simulink model "HEV_Simu_V1_1b"  (R2018a)
settings: Solver=ode23s  StartTime=0.0  StopTime=660  FixedStep=0.001  EnableMultiTasking=on
PreLoadFcn:
  | HevSimuVccWs_V1_PreLoad
  | %プラントモデルのコールバック・プリロード関数のバス定義
  | HEVPlant_Ptbs_V1_BusInfo
  | Engine_MapMdl_Ptbs_V1_BusInfo
  | Motor_MapMdl_Ptbs_V1_BusInfo
StartFcn:
  | tic
StopFcn:
  | toc
  | disp(['実時間の' num2str(max(tout)/toc) '倍速'])
model workspace (MAT data in the model file):
  Var = 0
undefined symbols (not defined in the file or in its folder): canChannel
libraries: canmsglib x108, canlib x35, simulink x2
(part 6 of 8)

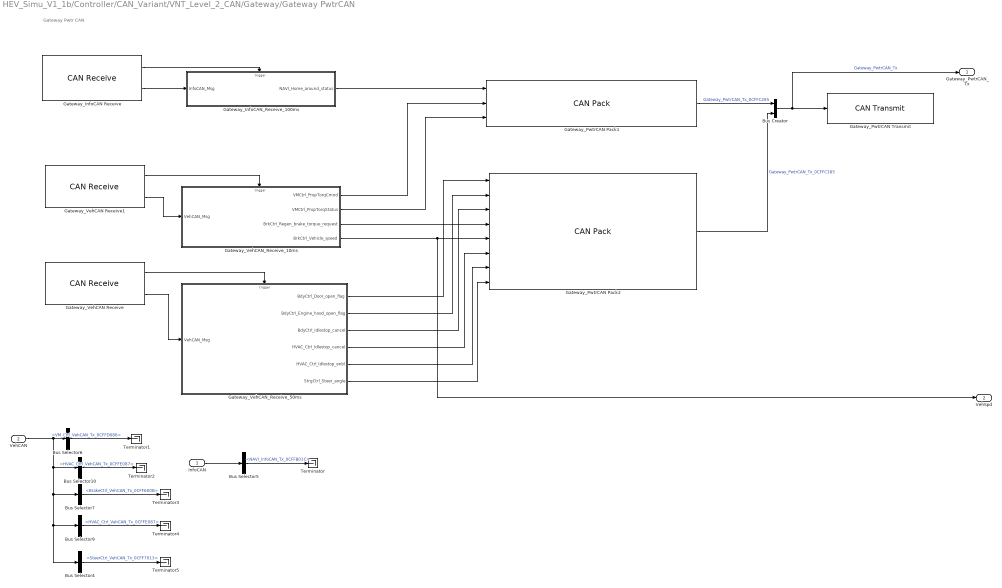
== system HEV_Simu_V1_1b/Controller/CAN_Variant/VNT_Level_2_CAN/Gateway/Gateway PwtrCAN ==
  note: Gateway Pwtr CAN
  InfoCAN : Inport
  VehCAN : Inport  Port=2
  Bus Creator : BusCreator  Inputs=2
  Bus Selector10 : BusSelector  OutputSignals=HVAC_Ctrl_VehCAN_Tx_0CFFE087
  Bus Selector4 : BusSelector  OutputSignals=SteerCtrl_VehCAN_Tx_0CFF7013
  Bus Selector5 : BusSelector  OutputSignals=NAVI_InfoCAN_Tx_0CFFB01C
  Bus Selector6 : BusSelector  OutputSignals=VM_Ctrl_VehCAN_Tx_0CFFD086
  Bus Selector7 : BusSelector  OutputSignals=BrakeCtrl_VehCAN_Tx_0CFF600B
  Bus Selector9 : BusSelector  OutputSignals=HVAC_Ctrl_VehCAN_Tx_0CFFE087
  Gateway_InfoCAN Receive : canlib/CAN Receive  BlockHandle=676.0001  DeviceMenu=MathWorks Virtual 1 (Channel 1)  Device=MathWorks Virtual 1 (Channel 1)  ObjConstructor=canChannel('MathWorks','Virtual 1',1)  EnableStandardIDsFilter=off  StandardIDs=0  EnableExtendedIDsFilter=off  ExtendedIDs=0  SampleTime=0.1  MsgsPerTimestep=all  StdIDsCombo=Allow all  ExtIDsCombo=Allow all  InternalFilterUpdateStatus=on  BusOutput=off
      settings: AttributesFormatString=<SampleTime = %<SampleTime>>  SourceProductName=Vehicle Network Toolbox  SourceProductBaseCode=VN
  Gateway_InfoCAN_Receive_100ms : Subsystem
  Gateway_PwtrCAN Pack1 : canmsglib/CAN Pack  CANdbFile=HEV_CANDB.dbc  MsgList=Gateway_PwtrCAN_Tx_1  MsgName=Gateway_PwtrCAN_Tx_1  MsgIDType=Extended (29-bit identifier)  MsgIdentifier=218088069  MsgLength=8  SignalInfo=NAVI_Home_around_status_G$0$16$1$2$1$0$1$0$0$65535$#VMCtrl_PropTorqCmnd_G$24$16$1$1$1$0$1.000000e-02$0$-300$300$#VMCtrl_PropTorqStatus_G$16$8$1$2$1$0$1$0$0$7$#  NSignals=3  StartBits=str2num('[int32(0);int32(24);int32(16)]')  SignalSizes=str2num('[int32(16);int32(16);int32(8)]')  ByteOrders=str2num('[int32(1);int32(1);int32(1)]')  DataTypes=str2num('[int32(2);int32(1);int32(2)]')  MultiplexTypes=str2num('[int32(1);int32(1);int32(1)]')  MultiplexValues=str2num('[double(0);double(0);double(0)]')  Factors=str2num('[double(1);double(1.000000e-02);double(1)]')  Offsets=str2num('[double(0);double(0);double(0)]')  Minimums=str2num('[double(0);double(-300);double(0)]')  Maximums=str2num('[double(65535);double(300);double(7)]')  Remote=off  ApplyMinMax=off  BusOutput=off
      settings: AttributesFormatString=<CANdbFile = %<CANdbFile>>  SourceProductName=Simulink Real-Time  SourceProductBaseCode=XP  DataFormat=CANdb specified signals
  Gateway_PwtrCAN Pack2 : canmsglib/CAN Pack  CANdbFile=HEV_CANDB.dbc  MsgList=Gateway_PwtrCAN_Tx_2  MsgName=Gateway_PwtrCAN_Tx_2  MsgIDType=Extended (29-bit identifier)  MsgIdentifier=218088325  MsgLength=8  SignalInfo=BdyCtrl_Door_open_flag_G$60$1$1$2$1$0$1$0$0$1$#BdyCtrl_Engine_hood_open_flg_G$59$1$1$2$1$0$1$0$0$1$#BdyCtrl_Idlestop_cancel_G$58$1$1$2$1$0$1$0$0$1$#BrkCtrl_Regen_brake_torque_re_G$16$16$1$1$1$0$1.000000e-02$0$-300$300$#BrkCtrl_Vehicle_speed_G$0$16$1$2$1$0$1.000000e-01$0$0$180$#HVAC_Ctrl_Idlestop_cancel_G$57$1$1$2$1$0$1$0$0$1$#HVAC_Ctrl_Idlestop_enbl_G$56$1$1$2$1$0$1$0$0$1$#StrgCtrl_Steer_angle_G$32$16$1$1$1$0$3.125000e-02$0$-720$720$#  NSignals=8  StartBits=str2num('[int32(60);int32(59);int32(58);int32(16);int32(0);int32(57);int32(56);int32(32)]')  SignalSizes=str2num('[int32(1);int32(1);int32(1);int32(16);int32(16);int32(1);int32(1);int32(16)]')  ByteOrders=str2num('[int32(1);int32(1);int32(1);int32(1);int32(1);int32(1);int32(1);int32(1)]')  DataTypes=str2num('[int32(2);int32(2);int32(2);int32(1);int32(2);int32(2);int32(2);int32(1)]')  MultiplexTypes=str2num('[int32(1);int32(1);int32(1);int32(1);int32(1);int32(1);int32(1);int32(1)]')  MultiplexValues=str2num('[double(0);double(0);double(0);double(0);double(0);double(0);double(0);double(0)]')  Factors=str2num('[double(1);double(1);double(1);double(1.000000e-02);double(1.000000e-01);double(1);double(1);double(3.125000e-02)]')  Offsets=str2num('[double(0);double(0);double(0);double(0);double(0);double(0);double(0);double(0)]')  Minimums=str2num('[double(0);double(0);double(0);double(-300);double(0);double(0);double(0);double(-720)]')  Maximums=str2num('[double(1);double(1);double(1);double(300);double(180);double(1);double(1);double(720)]')  Remote=off  ApplyMinMax=off  BusOutput=off
      settings: AttributesFormatString=<CANdbFile = %<CANdbFile>>  SourceProductName=Simulink Real-Time  SourceProductBaseCode=XP  DataFormat=CANdb specified signals
  Gateway_PwtrCAN Transmit : canlib/CAN Transmit  BlockHandle=688.0001  DeviceMenu=MathWorks Virtual 1 (Channel 1)  Device=MathWorks Virtual 1 (Channel 1)  ObjConstructor=canChannel('MathWorks','Virtual 1',1)  EnablePeriodicTransmit=on  MessagePeriod=0.01
      settings: AttributesFormatString=<MessagePeriod = %<MessagePeriod>>  SourceProductName=Vehicle Network Toolbox  SourceProductBaseCode=VN
  Gateway_VehCAN Receive : canlib/CAN Receive  BlockHandle=689.0001  DeviceMenu=MathWorks Virtual 1 (Channel 1)  Device=MathWorks Virtual 1 (Channel 1)  ObjConstructor=canChannel('MathWorks','Virtual 1',1)  EnableStandardIDsFilter=off  StandardIDs=0  EnableExtendedIDsFilter=off  ExtendedIDs=0  SampleTime=0.05  MsgsPerTimestep=all  StdIDsCombo=Allow all  ExtIDsCombo=Allow all  InternalFilterUpdateStatus=on  BusOutput=off
      settings: AttributesFormatString=<SampleTime = %<SampleTime>>  SourceProductName=Vehicle Network Toolbox  SourceProductBaseCode=VN
  Gateway_VehCAN Receive1 : canlib/CAN Receive  BlockHandle=690.0001  DeviceMenu=MathWorks Virtual 1 (Channel 1)  Device=MathWorks Virtual 1 (Channel 1)  ObjConstructor=canChannel('MathWorks','Virtual 1',1)  EnableStandardIDsFilter=off  StandardIDs=0  EnableExtendedIDsFilter=off  ExtendedIDs=0  SampleTime=0.01  MsgsPerTimestep=all  StdIDsCombo=Allow all  ExtIDsCombo=Allow all  InternalFilterUpdateStatus=on  BusOutput=off
      settings: AttributesFormatString=<SampleTime = %<SampleTime>>  SourceProductName=Vehicle Network Toolbox  SourceProductBaseCode=VN
  Gateway_VehCAN_Receive_10ms : Subsystem
  Gateway_VehCAN_Receive_50ms : Subsystem
  Terminator{,1..5} (6 alike) : Terminator
  Gateway_PwtrCAN_Tx : Outport
  VehSpd : Outport  Port=2
  wires:
  InfoCAN/1 -> Bus Selector5/1
  Bus Selector5/1 -> Terminator/1  "<NAVI_InfoCAN_Tx_0CFFB01C>"
  Gateway_InfoCAN_Receive_100ms/1(NAVI_Home_around_status) -> Gateway_PwtrCAN Pack1/1
  Gateway_InfoCAN Receive/2 -> Gateway_InfoCAN_Receive_100ms/1(InfoCAN_Msg)
  Gateway_InfoCAN Receive/1 -> Gateway_InfoCAN_Receive_100ms/Trigger
  VehCAN/1 -> Bus Selector10/1, Bus Selector7/1, Bus Selector4/1, Bus Selector9/1, Bus Selector6/1
  Bus Selector4/1 -> Terminator5/1  "<SteerCtrl_VehCAN_Tx_0CFF7013>"
  Bus Selector9/1 -> Terminator4/1  "<HVAC_Ctrl_VehCAN_Tx_0CFFE087>"
  Bus Selector7/1 -> Terminator3/1  "<BrakeCtrl_VehCAN_Tx_0CFF600B>"
  Bus Selector6/1 -> Terminator1/1  "<VM_Ctrl_VehCAN_Tx_0CFFD086>"
  Gateway_VehCAN Receive1/2 -> Gateway_VehCAN_Receive_10ms/1(VehCAN_Msg)
  Gateway_VehCAN_Receive_10ms/2(VMCtrl_PropTorqStatus) -> Gateway_PwtrCAN Pack1/3
  Gateway_VehCAN_Receive_10ms/1(VMCtrl_PropTorqCmnd) -> Gateway_PwtrCAN Pack1/2
  Gateway_VehCAN_Receive_10ms/4(BrkCtrl_Vehicle_speed) -> VehSpd/1, Gateway_PwtrCAN Pack2/5
  Gateway_VehCAN_Receive_10ms/3(BrkCtrl_Regen_brake_torque_request) -> Gateway_PwtrCAN Pack2/4
  Gateway_VehCAN Receive1/1 -> Gateway_VehCAN_Receive_10ms/Trigger
  Bus Selector10/1 -> Terminator2/1  "<HVAC_Ctrl_VehCAN_Tx_0CFFE087>"
  Gateway_VehCAN_Receive_50ms/6(StrgCtrl_Steer_angle) -> Gateway_PwtrCAN Pack2/8
  Gateway_VehCAN_Receive_50ms/5(HVAC_Ctrl_Idlestop_enbl) -> Gateway_PwtrCAN Pack2/7
  Gateway_VehCAN_Receive_50ms/4(HVAC_Ctrl_Idlestop_cancel) -> Gateway_PwtrCAN Pack2/6
  Gateway_VehCAN_Receive_50ms/3(BdyCtrl_Idlestop_cancel) -> Gateway_PwtrCAN Pack2/3
  Gateway_VehCAN_Receive_50ms/2(BdyCtrl_Engine_hood_open_flag) -> Gateway_PwtrCAN Pack2/2
  Gateway_VehCAN_Receive_50ms/1(BdyCtrl_Door_open_flag) -> Gateway_PwtrCAN Pack2/1
  Gateway_VehCAN Receive/2 -> Gateway_VehCAN_Receive_50ms/1(VehCAN_Msg)
  Gateway_VehCAN Receive/1 -> Gateway_VehCAN_Receive_50ms/Trigger
  Gateway_PwtrCAN Pack2/1 -> Bus Creator/2  "Gateway_PwtrCAN_Tx_0CFFC385"
  Gateway_PwtrCAN Pack1/1 -> Bus Creator/1  "Gateway_PwtrCAN_Tx_0CFFC285"
  Bus Creator/1 -> Gateway_PwtrCAN Transmit/1, Gateway_PwtrCAN_Tx/1  "Gateway_PwtrCAN_Tx"

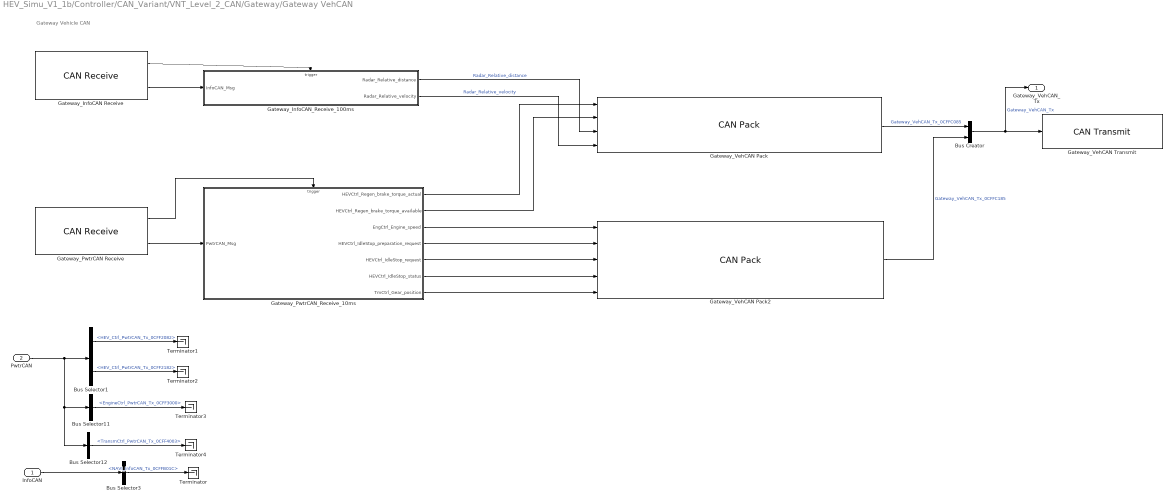
== system HEV_Simu_V1_1b/Controller/CAN_Variant/VNT_Level_2_CAN/Gateway/Gateway VehCAN ==
  note: Gateway Vehicle CAN
  InfoCAN : Inport
  PwtrCAN : Inport  Port=2
  Bus Creator : BusCreator  Inputs=2
  Bus Selector1 : BusSelector  OutputSignals=HEV_Ctrl_PwtrCAN_Tx_0CFF2082,HEV_Ctrl_PwtrCAN_Tx_0CFF2182
  Bus Selector11 : BusSelector  OutputSignals=EngineCtrl_PwtrCAN_Tx_0CFF3000
  Bus Selector12 : BusSelector  OutputSignals=TransmCtrl_PwtrCAN_Tx_0CFF4003
  Bus Selector3 : BusSelector  OutputSignals=NAVI_InfoCAN_Tx_0CFFB01C
  Gateway_InfoCAN Receive : canlib/CAN Receive  BlockHandle=791.0001  DeviceMenu=MathWorks Virtual 1 (Channel 1)  Device=MathWorks Virtual 1 (Channel 1)  ObjConstructor=canChannel('MathWorks','Virtual 1',1)  EnableStandardIDsFilter=off  StandardIDs=0  EnableExtendedIDsFilter=off  ExtendedIDs=0  SampleTime=0.1  MsgsPerTimestep=all  StdIDsCombo=Allow all  ExtIDsCombo=Allow all  InternalFilterUpdateStatus=on  BusOutput=off
      settings: AttributesFormatString=<SampleTime = %<SampleTime>>  SourceProductName=Vehicle Network Toolbox  SourceProductBaseCode=VN
  Gateway_InfoCAN_Receive_100ms : Subsystem
  Gateway_PwtrCAN Receive : canlib/CAN Receive  BlockHandle=801.0001  DeviceMenu=MathWorks Virtual 1 (Channel 1)  Device=MathWorks Virtual 1 (Channel 1)  ObjConstructor=canChannel('MathWorks','Virtual 1',1)  EnableStandardIDsFilter=off  StandardIDs=0  EnableExtendedIDsFilter=off  ExtendedIDs=0  SampleTime=0.01  MsgsPerTimestep=all  StdIDsCombo=Allow all  ExtIDsCombo=Allow all  InternalFilterUpdateStatus=on  BusOutput=off
      settings: AttributesFormatString=<SampleTime = %<SampleTime>>  SourceProductName=Vehicle Network Toolbox  SourceProductBaseCode=VN
  Gateway_PwtrCAN_Receive_10ms : Subsystem
  Gateway_VehCAN Pack : canmsglib/CAN Pack  CANdbFile=HEV_CANDB.dbc  MsgList=Gateway_VehCAN_Tx_1  MsgName=Gateway_VehCAN_Tx_1  MsgIDType=Extended (29-bit identifier)  MsgIdentifier=218087557  MsgLength=8  SignalInfo=HEVCtrl_Regen_brake_torque_act_G$48$16$1$1$1$0$6.250000e-02$0$-300$3000$#HEVCtrl_Regen_brake_torque_ave_G$32$16$1$1$1$0$6.250000e-02$0$-300$3000$#Radar_Relative_distance_G$0$16$1$2$1$0$1.000000e-02$0$0$500$#Radar_Relative_velocity_G$16$16$1$1$1$0$1.000000e-02$0$-50$50$#  NSignals=4  StartBits=str2num('[int32(48);int32(32);int32(0);int32(16)]')  SignalSizes=str2num('[int32(16);int32(16);int32(16);int32(16)]')  ByteOrders=str2num('[int32(1);int32(1);int32(1);int32(1)]')  DataTypes=str2num('[int32(1);int32(1);int32(2);int32(1)]')  MultiplexTypes=str2num('[int32(1);int32(1);int32(1);int32(1)]')  MultiplexValues=str2num('[double(0);double(0);double(0);double(0)]')  Factors=str2num('[double(6.250000e-02);double(6.250000e-02);double(1.000000e-02);double(1.000000e-02)]')  Offsets=str2num('[double(0);double(0);double(0);double(0)]')  Minimums=str2num('[double(-300);double(-300);double(0);double(-50)]')  Maximums=str2num('[double(3000);double(3000);double(500);double(50)]')  Remote=off  ApplyMinMax=off  BusOutput=off
      settings: AttributesFormatString=<CANdbFile = %<CANdbFile>>  SourceProductName=Simulink Real-Time  SourceProductBaseCode=XP  DataFormat=CANdb specified signals
  Gateway_VehCAN Pack2 : canmsglib/CAN Pack  CANdbFile=HEV_CANDB.dbc  MsgList=Gateway_VehCAN_Tx_2  MsgName=Gateway_VehCAN_Tx_2  MsgIDType=Extended (29-bit identifier)  MsgIdentifier=218087813  MsgLength=8  SignalInfo=EngCtrl_Engine_speed_G$0$16$1$2$1$0$1.250000e-01$0$0$8192$#HEV_IdleStopCtrl_preparation_r_G$24$1$1$2$1$0$1$0$0$1$#HEV_IdleStopCtrl_request_G$25$1$1$2$1$0$1$0$0$1$#HEV_IdleStopCtrl_status_G$26$1$1$2$1$0$1$0$0$1$#TmCtrl_Gear_position_G$16$8$1$2$1$0$1$0$0$5$#  NSignals=5  StartBits=str2num('[int32(0);int32(24);int32(25);int32(26);int32(16)]')  SignalSizes=str2num('[int32(16);int32(1);int32(1);int32(1);int32(8)]')  ByteOrders=str2num('[int32(1);int32(1);int32(1);int32(1);int32(1)]')  DataTypes=str2num('[int32(2);int32(2);int32(2);int32(2);int32(2)]')  MultiplexTypes=str2num('[int32(1);int32(1);int32(1);int32(1);int32(1)]')  MultiplexValues=str2num('[double(0);double(0);double(0);double(0);double(0)]')  Factors=str2num('[double(1.250000e-01);double(1);double(1);double(1);double(1)]')  Offsets=str2num('[double(0);double(0);double(0);double(0);double(0)]')  Minimums=str2num('[double(0);double(0);double(0);double(0);double(0)]')  Maximums=str2num('[double(8192);double(1);double(1);double(1);double(5)]')  Remote=off  ApplyMinMax=off  BusOutput=off
      settings: AttributesFormatString=<CANdbFile = %<CANdbFile>>  SourceProductName=Simulink Real-Time  SourceProductBaseCode=XP  DataFormat=CANdb specified signals
  Gateway_VehCAN Transmit : canlib/CAN Transmit  BlockHandle=840.0001  DeviceMenu=MathWorks Virtual 1 (Channel 1)  Device=MathWorks Virtual 1 (Channel 1)  ObjConstructor=canChannel('MathWorks','Virtual 1',1)  EnablePeriodicTransmit=on  MessagePeriod=0.05
      settings: AttributesFormatString=<MessagePeriod = %<MessagePeriod>>  SourceProductName=Vehicle Network Toolbox  SourceProductBaseCode=VN
  Terminator{,1..4} (5 alike) : Terminator
  Gateway_VehCAN_Tx : Outport
  wires:
  InfoCAN/1 -> Bus Selector3/1
  Bus Selector3/1 -> Terminator/1  "<NAVI_InfoCAN_Tx_0CFFB01C>"
  Gateway_InfoCAN Receive/2 -> Gateway_InfoCAN_Receive_100ms/1(InfoCAN_Msg)
  Gateway_InfoCAN Receive/1 -> Gateway_InfoCAN_Receive_100ms/Trigger
  Gateway_InfoCAN_Receive_100ms/2(Radar_Relative_velocity) -> Gateway_VehCAN Pack/4  "Radar_Relative_velocity"
  Gateway_InfoCAN_Receive_100ms/1(Radar_Relative_distance) -> Gateway_VehCAN Pack/3  "Radar_Relative_distance"
  Bus Creator/1 -> Gateway_VehCAN Transmit/1, Gateway_VehCAN_Tx/1  "Gateway_VehCAN_Tx"
  Gateway_VehCAN Pack2/1 -> Bus Creator/2  "Gateway_VehCAN_Tx_0CFFC185"
  Gateway_VehCAN Pack/1 -> Bus Creator/1  "Gateway_VehCAN_Tx_0CFFC085"
  PwtrCAN/1 -> Bus Selector11/1, Bus Selector12/1, Bus Selector1/1
  Bus Selector1/1 -> Terminator1/1  "<HEV_Ctrl_PwtrCAN_Tx_0CFF2082>"
  Bus Selector1/2 -> Terminator2/1  "<HEV_Ctrl_PwtrCAN_Tx_0CFF2182>"
  Bus Selector11/1 -> Terminator3/1  "<EngineCtrl_PwtrCAN_Tx_0CFF3000>"
  Bus Selector12/1 -> Terminator4/1  "<TransmCtrl_PwtrCAN_Tx_0CFF4003>"
  Gateway_PwtrCAN_Receive_10ms/1(HEVCtrl_Regen_brake_torque_actual) -> Gateway_VehCAN Pack/1
  Gateway_PwtrCAN_Receive_10ms/2(HEVCtrl_Regen_brake_torque_available) -> Gateway_VehCAN Pack/2
  Gateway_PwtrCAN_Receive_10ms/3(EngCtrl_Engine_speed) -> Gateway_VehCAN Pack2/1
  Gateway_PwtrCAN_Receive_10ms/4(HEVCtrl_IdleStop_preparation_request) -> Gateway_VehCAN Pack2/2
  Gateway_PwtrCAN_Receive_10ms/5(HEVCtrl_IdleStop_request) -> Gateway_VehCAN Pack2/3
  Gateway_PwtrCAN_Receive_10ms/6(HEVCtrl_IdleStop_status) -> Gateway_VehCAN Pack2/4
  Gateway_PwtrCAN_Receive_10ms/7(TmCtrl_Gear_position) -> Gateway_VehCAN Pack2/5
  Gateway_PwtrCAN Receive/1 -> Gateway_PwtrCAN_Receive_10ms/Trigger
  Gateway_PwtrCAN Receive/2 -> Gateway_PwtrCAN_Receive_10ms/1(PwtrCAN_Msg)

== system HEV_Simu_V1_1b/Controller/CAN_Variant/VNT_Level_2_CAN/Gateway/Info Hub ==
  note: Info Hub
  InfoCAN : Inport
  VehCAN : Inport  Port=2
  PwtrCAN : Inport  Port=3
  Bus Creator3 : BusCreator  Inputs=3
  tag scope: CAN=scoped
  wires:
  PwtrCAN/1 -> Bus Creator3/3
  Bus Creator3/1 -> [CAN]
  VehCAN/1 -> Bus Creator3/2
  InfoCAN/1 -> Bus Creator3/1

== system HEV_Simu_V1_1b/Controller/CAN_Variant/VNT_Level_2_CAN/HEV_Ctrl/HEV_Ctrl_PwtrCAN Tx ==
  note: Function of CAN transmit
      | ・conversion fromCAN application signal to signal of CAN message
  note: HEV control
  note: CAN transmit
  HEV_Ctrl_PwtrCAN_Tx_Apli : Inport
  Bus Creator : BusCreator  Inputs=2
  Bus Selector1 : BusSelector  OutputSignals=HEVCtrl_Engine_torque_request,HEVCtrl_Motor_torque_request,HEVCtrl_Regen_brake_torque_actual,HEVCtrl_Regen_brake_torque_available,HEVCtrl_IdleStop_preparation_request,HEVCtrl_IdleStop_request,HEVCtrl_IdleStop_status
  HEV_Ctrl_PwtrCAN Pack : canmsglib/CAN Pack  CANdbFile=HEV_CANDB.dbc  MsgList=HEV_Ctrl_PwtrCAN_Tx_1  MsgName=HEV_Ctrl_PwtrCAN_Tx_1  MsgIDType=Extended (29-bit identifier)  MsgIdentifier=218046594  MsgLength=8  SignalInfo=HEVCtrl_Engine_torque_request$0$16$1$1$1$0$1.562500e-02$0$-300$300$#HEVCtrl_Motor_torque_request$16$16$1$1$1$0$1.562500e-02$0$-300$300$#HEVCtrl_Regen_brake_torque_actua$48$16$1$1$1$0$6.250000e-02$0$-300$3000$#HEVCtrl_Regen_brake_torque_avail$32$16$1$1$1$0$6.250000e-02$0$-300$3000$#  NSignals=4  StartBits=str2num('[int32(0);int32(16);int32(48);int32(32)]')  SignalSizes=str2num('[int32(16);int32(16);int32(16);int32(16)]')  ByteOrders=str2num('[int32(1);int32(1);int32(1);int32(1)]')  DataTypes=str2num('[int32(1);int32(1);int32(1);int32(1)]')  MultiplexTypes=str2num('[int32(1);int32(1);int32(1);int32(1)]')  MultiplexValues=str2num('[double(0);double(0);double(0);double(0)]')  Factors=str2num('[double(1.562500e-02);double(1.562500e-02);double(6.250000e-02);double(6.250000e-02)]')  Offsets=str2num('[double(0);double(0);double(0);double(0)]')  Minimums=str2num('[double(-300);double(-300);double(-300);double(-300)]')  Maximums=str2num('[double(300);double(300);double(3000);double(3000)]')  Remote=off  ApplyMinMax=off  BusOutput=off
      settings: AttributesFormatString=<CANdbFile = %<CANdbFile>>  SourceProductName=Simulink Real-Time  SourceProductBaseCode=XP  DataFormat=CANdb specified signals
  HEV_Ctrl_PwtrCAN Pack2 : canmsglib/CAN Pack  CANdbFile=HEV_CANDB.dbc  MsgList=HEV_Ctrl_PwtrCAN_Tx_2  MsgName=HEV_Ctrl_PwtrCAN_Tx_2  MsgIDType=Extended (29-bit identifier)  MsgIdentifier=218046850  MsgLength=8  SignalInfo=HEV_IdleStopCtrl_preparation_req$0$1$1$2$1$0$1$0$0$1$#HEV_IdleStopCtrl_request$1$1$1$2$1$0$1$0$0$1$#HEV_IdleStopCtrl_status$2$1$1$2$1$0$1$0$0$1$#  NSignals=3  StartBits=str2num('[int32(0);int32(1);int32(2)]')  SignalSizes=str2num('[int32(1);int32(1);int32(1)]')  ByteOrders=str2num('[int32(1);int32(1);int32(1)]')  DataTypes=str2num('[int32(2);int32(2);int32(2)]')  MultiplexTypes=str2num('[int32(1);int32(1);int32(1)]')  MultiplexValues=str2num('[double(0);double(0);double(0)]')  Factors=str2num('[double(1);double(1);double(1)]')  Offsets=str2num('[double(0);double(0);double(0)]')  Minimums=str2num('[double(0);double(0);double(0)]')  Maximums=str2num('[double(1);double(1);double(1)]')  Remote=off  ApplyMinMax=off  BusOutput=off
      settings: AttributesFormatString=<CANdbFile = %<CANdbFile>>  SourceProductName=Simulink Real-Time  SourceProductBaseCode=XP  DataFormat=CANdb specified signals
  HEV_Ctrl_PwtrCAN Transmit : canlib/CAN Transmit  BlockHandle=923.0001  DeviceMenu=MathWorks Virtual 1 (Channel 1)  Device=MathWorks Virtual 1 (Channel 1)  ObjConstructor=canChannel('MathWorks','Virtual 1',1)  EnablePeriodicTransmit=on  MessagePeriod=0.01
      settings: AttributesFormatString=<MessagePeriod = %<MessagePeriod>>  SourceProductName=Vehicle Network Toolbox  SourceProductBaseCode=VN
  HEV_Ctrl_PwtrCAN_Tx : Outport
  wires:
  Bus Selector1/2 -> HEV_Ctrl_PwtrCAN Pack/2  "<HEVCtrl_Motor_torque_request>"
  Bus Selector1/1 -> HEV_Ctrl_PwtrCAN Pack/1  "<HEVCtrl_Engine_torque_request>"
  Bus Selector1/3 -> HEV_Ctrl_PwtrCAN Pack/3  "<HEVCtrl_Regen_brake_torque_actual>"
  Bus Selector1/6 -> HEV_Ctrl_PwtrCAN Pack2/2  "<HEVCtrl_IdleStop_request>"
  Bus Selector1/4 -> HEV_Ctrl_PwtrCAN Pack/4  "<HEVCtrl_Regen_brake_torque_available>"
  Bus Selector1/5 -> HEV_Ctrl_PwtrCAN Pack2/1  "<HEVCtrl_IdleStop_preparation_request>"
  HEV_Ctrl_PwtrCAN Pack2/1 -> Bus Creator/2  "HEV_Ctrl_PwtrCAN_Tx_0CFF2182"
  HEV_Ctrl_PwtrCAN Pack/1 -> Bus Creator/1  "HEV_Ctrl_PwtrCAN_Tx_0CFF2082"
  Bus Selector1/7 -> HEV_Ctrl_PwtrCAN Pack2/3  "<HEVCtrl_IdleStop_status>"
  Bus Creator/1 -> HEV_Ctrl_PwtrCAN Transmit/1, HEV_Ctrl_PwtrCAN_Tx/1  "HEV_Ctrl_PwtrCAN_Tx"
  HEV_Ctrl_PwtrCAN_Tx_Apli/1 -> Bus Selector1/1

== system HEV_Simu_V1_1b/Controller/CAN_Variant/VNT_Level_2_CAN/HEV_Ctrl/HEV_Ctrl_PwtrCAN_Rx ==
  note: Function of CAN receive
      | ・CAN message selection
      | ・conversion from CAN signal to CAN application signal with bus object
  note: HEV control
  note: CAN receive
  PwtrCAN : Inport
  Bus Creator1 : BusCreator  Inputs=13  OutDataTypeStr=Bus: HEV_Ctrl_PwtrCAN_Rx_Bus
  Bus Selector2 : BusSelector  OutputSignals=EngineCtrl_PwtrCAN_Tx_0CFF3000
  Bus Selector4 : BusSelector  OutputSignals=TransmCtrl_PwtrCAN_Tx_0CFF4003
  Bus Selector5 : BusSelector  OutputSignals=MotorCtrl_PwtrCAN_Tx_0CFF5083
  Bus Selector6 : BusSelector  OutputSignals=BatteryCtrl_PwtrCAN_Tx_0CFF8084
  Bus Selector7 : BusSelector  OutputSignals=Gateway_PwtrCAN_Tx_0CFFC385,Gateway_PwtrCAN_Tx_0CFFC285
  HEV_Ctrl_PwtrCAN Receive : canlib/CAN Receive  BlockHandle=949.0001  DeviceMenu=MathWorks Virtual 1 (Channel 1)  Device=MathWorks Virtual 1 (Channel 1)  ObjConstructor=canChannel('MathWorks','Virtual 1',1)  EnableStandardIDsFilter=off  StandardIDs=0  EnableExtendedIDsFilter=off  ExtendedIDs=0  SampleTime=0.01  MsgsPerTimestep=all  StdIDsCombo=Allow all  ExtIDsCombo=Allow all  InternalFilterUpdateStatus=on  BusOutput=off
      settings: AttributesFormatString=<SampleTime = %<SampleTime>>  SourceProductName=Vehicle Network Toolbox  SourceProductBaseCode=VN
  HEV_Ctrl_PwtrCAN Receive1 : canlib/CAN Receive  BlockHandle=950.0001  DeviceMenu=MathWorks Virtual 1 (Channel 1)  Device=MathWorks Virtual 1 (Channel 1)  ObjConstructor=canChannel('MathWorks','Virtual 1',1)  EnableStandardIDsFilter=off  StandardIDs=0  EnableExtendedIDsFilter=off  ExtendedIDs=0  SampleTime=0.05  MsgsPerTimestep=all  StdIDsCombo=Allow all  ExtIDsCombo=Allow all  InternalFilterUpdateStatus=on  BusOutput=off
      settings: AttributesFormatString=<SampleTime = %<SampleTime>>  SourceProductName=Vehicle Network Toolbox  SourceProductBaseCode=VN
  HEV_Ctrl_PwtrCAN_Receive_10ms : Subsystem
  HEV_Ctrl_PwtrCAN_Receive_50ms : Subsystem
  Rate Transition1 : RateTransition  Deterministic=off
      settings: AttributesFormatString=<Deterministic=%<Deterministic>>
  Terminator{,1..5} (6 alike) : Terminator
  HEV_Ctrl_PwtrCAN_Rx : Outport
  wires:
  PwtrCAN/1 -> Bus Selector2/1, Bus Selector5/1, Bus Selector4/1, Bus Selector6/1, Bus Selector7/1
  Bus Creator1/1 -> Rate Transition1/1
  Rate Transition1/1 -> HEV_Ctrl_PwtrCAN_Rx/1  "HEV_Ctrl_PwtrCAN_Rx"
  Bus Selector7/2 -> Terminator1/1  "<Gateway_PwtrCAN_Tx_0CFFC285>"
  Bus Selector6/1 -> Terminator2/1  "<BatteryCtrl_PwtrCAN_Tx_0CFF8084>"
  HEV_Ctrl_PwtrCAN_Receive_50ms/1(BatCtrl_SOC) -> Bus Creator1/1
  HEV_Ctrl_PwtrCAN_Receive_50ms/2(VMCtrl_PropTorqStatus) -> Bus Creator1/11
  HEV_Ctrl_PwtrCAN_Receive_50ms/3(VMCtrl_PropTorqCmnd) -> Bus Creator1/12
  HEV_Ctrl_PwtrCAN_Receive_50ms/4(NAVI_Home_around_status) -> Bus Creator1/13
  Bus Selector7/1 -> Terminator/1  "<Gateway_PwtrCAN_Tx_0CFFC385>"
  Bus Selector4/1 -> Terminator3/1  "<TransmCtrl_PwtrCAN_Tx_0CFF4003>"
  Bus Selector5/1 -> Terminator4/1  "<MotorCtrl_PwtrCAN_Tx_0CFF5083>"
  Bus Selector2/1 -> Terminator5/1  "<EngineCtrl_PwtrCAN_Tx_0CFF3000>"
  HEV_Ctrl_PwtrCAN_Receive_10ms/1(TmCtrl_Clutch_position) -> Bus Creator1/2
  HEV_Ctrl_PwtrCAN_Receive_10ms/2(TmCtrl_Gear_position) -> Bus Creator1/3
  HEV_Ctrl_PwtrCAN_Receive_10ms/3(BrkCtrl_Vehicle_speed) -> Bus Creator1/4
  HEV_Ctrl_PwtrCAN_Receive_10ms/4(BrkCtrl_Regen_brake_torque_request) -> Bus Creator1/5
  HEV_Ctrl_PwtrCAN_Receive_10ms/5(MtrCtrl_Motor_torque_actual) -> Bus Creator1/6
  HEV_Ctrl_PwtrCAN_Receive_10ms/6(MtrCtrl_Motor_torque_available) -> Bus Creator1/7
  HEV_Ctrl_PwtrCAN_Receive_10ms/7(MtrCtrl_Motor_regen_torque_available) -> Bus Creator1/8
  HEV_Ctrl_PwtrCAN_Receive_10ms/8(EngCtrl_Engine_speed) -> Bus Creator1/9
  HEV_Ctrl_PwtrCAN_Receive_10ms/9(EngCtrl_Engine_torque_actual) -> Bus Creator1/10
  HEV_Ctrl_PwtrCAN Receive/1 -> HEV_Ctrl_PwtrCAN_Receive_10ms/Trigger
  HEV_Ctrl_PwtrCAN Receive1/1 -> HEV_Ctrl_PwtrCAN_Receive_50ms/Trigger
  HEV_Ctrl_PwtrCAN Receive1/2 -> HEV_Ctrl_PwtrCAN_Receive_50ms/1(PwtrCAN_Msg)
  HEV_Ctrl_PwtrCAN Receive/2 -> HEV_Ctrl_PwtrCAN_Receive_10ms/1(PwtrCAN_Msg)

== system HEV_Simu_V1_1b/Controller/CAN_Variant/VNT_Level_2_CAN/HVAC_Ctrl/HVAC_Ctrl_VehCAN Tx ==
  note: HVAC Control
  note: Function of CAN transmit
      | ・conversion fromCAN application signal to signal of CAN message
  note: CAN transmit
  HVAC_Ctrl_VehCAN_Tx_Apli : Inport
  Bus Creator1 : BusCreator  Inputs=1
  Bus Selector2 : BusSelector  OutputSignals=HVAC_Ctrl_Idlestop_cancel,HVAC_Ctrl_Idlestop_enbl
  HVAC_Ctrl_VehCAN Pack : canmsglib/CAN Pack  CANdbFile=HEV_CANDB.dbc  MsgList=HVAC_Ctrl_VehCAN_Tx  MsgName=HVAC_Ctrl_VehCAN_Tx  MsgIDType=Extended (29-bit identifier)  MsgIdentifier=218095751  MsgLength=8  SignalInfo=HVAC_Ctrl_Idlestop_cancel$1$1$1$2$1$0$1$0$0$1$#HVAC_Ctrl_Idlestop_enbl$0$1$1$2$1$0$1$0$0$1$#  NSignals=2  StartBits=str2num('[int32(1);int32(0)]')  SignalSizes=str2num('[int32(1);int32(1)]')  ByteOrders=str2num('[int32(1);int32(1)]')  DataTypes=str2num('[int32(2);int32(2)]')  MultiplexTypes=str2num('[int32(1);int32(1)]')  MultiplexValues=str2num('[double(0);double(0)]')  Factors=str2num('[double(1);double(1)]')  Offsets=str2num('[double(0);double(0)]')  Minimums=str2num('[double(0);double(0)]')  Maximums=str2num('[double(1);double(1)]')  Remote=off  ApplyMinMax=off  BusOutput=off
      settings: AttributesFormatString=<CANdbFile = %<CANdbFile>>  SourceProductName=Simulink Real-Time  SourceProductBaseCode=XP  DataFormat=CANdb specified signals
  HVAC_Ctrl_VehCAN Transmit : canlib/CAN Transmit  BlockHandle=1100.0001  DeviceMenu=MathWorks Virtual 1 (Channel 1)  Device=MathWorks Virtual 1 (Channel 1)  ObjConstructor=canChannel('MathWorks','Virtual 1',1)  EnablePeriodicTransmit=on  MessagePeriod=0.05
      settings: AttributesFormatString=<MessagePeriod = %<MessagePeriod>>  SourceProductName=Vehicle Network Toolbox  SourceProductBaseCode=VN
  HVAC_Ctrl_VehCAN_Tx : Outport
  wires:
  Bus Selector2/2 -> HVAC_Ctrl_VehCAN Pack/2  "<HVAC_Ctrl_Idlestop_enbl>"
  Bus Selector2/1 -> HVAC_Ctrl_VehCAN Pack/1  "<HVAC_Ctrl_Idlestop_cancel>"
  HVAC_Ctrl_VehCAN Pack/1 -> HVAC_Ctrl_VehCAN Transmit/1, Bus Creator1/1  "HVAC_Ctrl_VehCAN_Tx_0CFFE087"
  HVAC_Ctrl_VehCAN_Tx_Apli/1 -> Bus Selector2/1
  Bus Creator1/1 -> HVAC_Ctrl_VehCAN_Tx/1  "HVAC_Ctrl_VehCAN_Tx"

== system HEV_Simu_V1_1b/Controller/CAN_Variant/VNT_Level_2_CAN/HVAC_Ctrl/HVAC_Ctrl_VehCAN_Rx ==
  note: HVAC Control
  note: Function of CAN receive
      | ・CAN message selection
      | ・conversion from CAN signal to CAN application signal with bus object
  note: CAN receive
  VehCAN : Inport
  Bus Creator : BusCreator  Inputs=3
  Bus Selector3 : BusSelector  OutputSignals=VM_Ctrl_VehCAN_Tx_0CFFD086
  HVAC_Ctrl_VehCAN Receive : canlib/CAN Receive  BlockHandle=1116.0001  DeviceMenu=MathWorks Virtual 1 (Channel 1)  Device=MathWorks Virtual 1 (Channel 1)  ObjConstructor=canChannel('MathWorks','Virtual 1',1)  EnableStandardIDsFilter=off  StandardIDs=0  EnableExtendedIDsFilter=off  ExtendedIDs=0  SampleTime=0.05  MsgsPerTimestep=all  StdIDsCombo=Allow all  ExtIDsCombo=Allow all  InternalFilterUpdateStatus=on  BusOutput=off
      settings: AttributesFormatString=<SampleTime = %<SampleTime>>  SourceProductName=Vehicle Network Toolbox  SourceProductBaseCode=VN
  HVAC_Ctrl_VehCAN_Receive_50ms : Subsystem
  Rate Transition1 : RateTransition  Deterministic=off
      settings: AttributesFormatString=<Deterministic=%<Deterministic>>
  Terminator : Terminator
  HVAC_Ctrl_VehCAN_Rx : Outport
  wires:
  Bus Creator/1 -> Rate Transition1/1
  VehCAN/1 -> Bus Selector3/1
  Rate Transition1/1 -> HVAC_Ctrl_VehCAN_Rx/1  "HVAC_Ctrl_VehCAN_Rx"
  Bus Selector3/1 -> Terminator/1  "<VM_Ctrl_VehCAN_Tx_0CFFD086>"
  HVAC_Ctrl_VehCAN_Receive_50ms/1(EngCtrl_Engine_speed) -> Bus Creator/1
  HVAC_Ctrl_VehCAN_Receive_50ms/2(HEVCtrl_IdleStop_preparation_request) -> Bus Creator/2
  HVAC_Ctrl_VehCAN_Receive_50ms/3(HEVCtrl_IdleStop_status) -> Bus Creator/3
  HVAC_Ctrl_VehCAN Receive/1 -> HVAC_Ctrl_VehCAN_Receive_50ms/Trigger
  HVAC_Ctrl_VehCAN Receive/2 -> HVAC_Ctrl_VehCAN_Receive_50ms/1(VehCAN_Msg)

== system HEV_Simu_V1_1b/Controller/CAN_Variant/VNT_Level_2_CAN/Motor_Ctrl/MotorCtrl_PwtrCAN Tx ==
  note: Function of CAN transmit
      | ・conversion fromCAN application signal to signal of CAN message
  note: Motor Control
  note: CAN transmit
  IMotorCtrl_PwtrCAN_Tx_Apli : Inport
  Bus Creator1 : BusCreator  Inputs=1
  Bus Selector1 : BusSelector  OutputSignals=MtrCtrl_Motor_regen_torque_available,MtrCtrl_Motor_torque_actual,MtrCtrl_Motor_torque_available
  MotorCtrl_PwtrCAN Pack : canmsglib/CAN Pack  CANdbFile=HEV_CANDB.dbc  MsgList=MotorCtrl_PwtrCAN_Tx  MsgName=MotorCtrl_PwtrCAN_Tx  MsgIDType=Extended (29-bit identifier)  MsgIdentifier=218058883  MsgLength=8  SignalInfo=MtrCtrl_Motor_regen_torque_avail$32$16$1$1$1$0$1.000000e-02$0$-300$300$#MtrCtrl_Motor_torque_actual$0$16$1$1$1$0$1.000000e-02$0$-300$300$#MtrCtrl_Motor_torque_available$16$16$1$1$1$0$1.000000e-02$0$-300$300$#  NSignals=3  StartBits=str2num('[int32(32);int32(0);int32(16)]')  SignalSizes=str2num('[int32(16);int32(16);int32(16)]')  ByteOrders=str2num('[int32(1);int32(1);int32(1)]')  DataTypes=str2num('[int32(1);int32(1);int32(1)]')  MultiplexTypes=str2num('[int32(1);int32(1);int32(1)]')  MultiplexValues=str2num('[double(0);double(0);double(0)]')  Factors=str2num('[double(1.000000e-02);double(1.000000e-02);double(1.000000e-02)]')  Offsets=str2num('[double(0);double(0);double(0)]')  Minimums=str2num('[double(-300);double(-300);double(-300)]')  Maximums=str2num('[double(300);double(300);double(300)]')  Remote=off  ApplyMinMax=off  BusOutput=off
      settings: AttributesFormatString=<CANdbFile = %<CANdbFile>>  SourceProductName=Simulink Real-Time  SourceProductBaseCode=XP  DataFormat=CANdb specified signals
  MotorCtrl_PwtrCAN Transmit : canlib/CAN Transmit  BlockHandle=1199.0001  DeviceMenu=MathWorks Virtual 1 (Channel 1)  Device=MathWorks Virtual 1 (Channel 1)  ObjConstructor=canChannel('MathWorks','Virtual 1',1)  EnablePeriodicTransmit=on  MessagePeriod=0.01
      settings: AttributesFormatString=<MessagePeriod = %<MessagePeriod>>  SourceProductName=Vehicle Network Toolbox  SourceProductBaseCode=VN
  MotorCtrl_PwtrCAN_Tx_0CFF5083 : Outport
  wires:
  Bus Selector1/2 -> MotorCtrl_PwtrCAN Pack/2  "<MtrCtrl_Motor_torque_actual>"
  Bus Creator1/1 -> MotorCtrl_PwtrCAN Transmit/1, MotorCtrl_PwtrCAN_Tx_0CFF5083/1  "MotorCtrl_PwtrCAN_Tx"
  Bus Selector1/3 -> MotorCtrl_PwtrCAN Pack/3  "<MtrCtrl_Motor_torque_available>"
  MotorCtrl_PwtrCAN Pack/1 -> Bus Creator1/1  "MotorCtrl_PwtrCAN_Tx_0CFF5083"
  IMotorCtrl_PwtrCAN_Tx_Apli/1 -> Bus Selector1/1
  Bus Selector1/1 -> MotorCtrl_PwtrCAN Pack/1  "<MtrCtrl_Motor_regen_torque_available>"

== system HEV_Simu_V1_1b/Controller/CAN_Variant/VNT_Level_2_CAN/Motor_Ctrl/MotorCtrl_PwtrCAN_Rx ==
  note: Function of CAN receive
      | ・CAN message selection
      | ・conversion from CAN signal to CAN application signal with bus object
  note: Motor Control
  note: CAN receive
  PwtrCAN : Inport
  Bus Creator7 : BusCreator  Inputs=3
  Bus Selector3 : BusSelector  OutputSignals=HEV_Ctrl_PwtrCAN_Tx_0CFF2082
  Bus Selector4 : BusSelector  OutputSignals=EngineCtrl_PwtrCAN_Tx_0CFF3000
  Bus Selector5 : BusSelector  OutputSignals=TransmCtrl_PwtrCAN_Tx_0CFF4003
  MotorCtrl_PwtrCAN Receive : canlib/CAN Receive  BlockHandle=1218.0001  DeviceMenu=MathWorks Virtual 1 (Channel 1)  Device=MathWorks Virtual 1 (Channel 1)  ObjConstructor=canChannel('MathWorks','Virtual 1',1)  EnableStandardIDsFilter=off  StandardIDs=0  EnableExtendedIDsFilter=off  ExtendedIDs=0  SampleTime=0.01  MsgsPerTimestep=all  StdIDsCombo=Allow all  ExtIDsCombo=Allow all  InternalFilterUpdateStatus=on  BusOutput=off
      settings: AttributesFormatString=<SampleTime = %<SampleTime>>  SourceProductName=Vehicle Network Toolbox  SourceProductBaseCode=VN
  MotorCtrl_PwtrCAN_Receive_10ms : Subsystem
  Rate Transition1 : RateTransition  Deterministic=off
      settings: AttributesFormatString=<Deterministic=%<Deterministic>>
  Terminator : Terminator
  Terminator1 : Terminator
  Terminator2 : Terminator
  MotorCtrl_PwtrCAN_Rx : Outport
  wires:
  PwtrCAN/1 -> Bus Selector4/1, Bus Selector3/1, Bus Selector5/1
  Bus Creator7/1 -> Rate Transition1/1
  Rate Transition1/1 -> MotorCtrl_PwtrCAN_Rx/1  "MotorCtrl_PwtrCAN_Rx"
  Bus Selector5/1 -> Terminator/1  "<TransmCtrl_PwtrCAN_Tx_0CFF4003>"
  Bus Selector3/1 -> Terminator1/1  "<HEV_Ctrl_PwtrCAN_Tx_0CFF2082>"
  Bus Selector4/1 -> Terminator2/1  "<EngineCtrl_PwtrCAN_Tx_0CFF3000>"
  MotorCtrl_PwtrCAN_Receive_10ms/1(TmCtrl_Clutch_position) -> Bus Creator7/1
  MotorCtrl_PwtrCAN_Receive_10ms/2(HEVCtrl_Motor_torque_request) -> Bus Creator7/2
  MotorCtrl_PwtrCAN_Receive_10ms/3(EngCtrl_Engine_speed) -> Bus Creator7/3
  MotorCtrl_PwtrCAN Receive/2 -> MotorCtrl_PwtrCAN_Receive_10ms/1(PwtrCAN_Msg)
  MotorCtrl_PwtrCAN Receive/1 -> MotorCtrl_PwtrCAN_Receive_10ms/Trigger

== system HEV_Simu_V1_1b/Controller/CAN_Variant/VNT_Level_2_CAN/NAVI/NAVI_CAN_Rx ==
  note: CAN receive
  note: Navigation
  InfoCAN : Inport
  Bus Creator : BusCreator  Inputs=1  OutDataTypeStr=Bus: NAVI_InfoCAN_Rx_Bus
      settings: AttributesFormatString=<%<OutDataTypeStr>>
  Bus Selector1 : BusSelector  OutputSignals=Gateway_InfoCAN_Tx_0CFFC485
  NAVI_InfoCAN Receive : canlib/CAN Receive  BlockHandle=1292.0001  DeviceMenu=MathWorks Virtual 1 (Channel 1)  Device=MathWorks Virtual 1 (Channel 1)  ObjConstructor=canChannel('MathWorks','Virtual 1',1)  EnableStandardIDsFilter=off  StandardIDs=0  EnableExtendedIDsFilter=off  ExtendedIDs=0  SampleTime=0.1  MsgsPerTimestep=all  StdIDsCombo=Allow all  ExtIDsCombo=Allow all  InternalFilterUpdateStatus=on  BusOutput=off
      settings: AttributesFormatString=<SampleTime = %<SampleTime>>  SourceProductName=Vehicle Network Toolbox  SourceProductBaseCode=VN
  NAVI_InfoCAN_Receive_100ms : Subsystem
  Rate Transition1 : RateTransition  Deterministic=off
      settings: AttributesFormatString=<Deterministic=%<Deterministic>>
  Terminator : Terminator
  NAVI_InfoCAN_Rx : Outport
  wires:
  Rate Transition1/1 -> NAVI_InfoCAN_Rx/1  "NAVI_InfoCAN_Rx"
  InfoCAN/1 -> Bus Selector1/1
  Bus Selector1/1 -> Terminator/1  "<Gateway_InfoCAN_Tx_0CFFC485>"
  NAVI_InfoCAN Receive/2 -> NAVI_InfoCAN_Receive_100ms/1(InfoCAN_Msg)
  NAVI_InfoCAN Receive/1 -> NAVI_InfoCAN_Receive_100ms/Trigger
  Bus Creator/1 -> Rate Transition1/1
  NAVI_InfoCAN_Receive_100ms/1(BrkCtrl_Vehicle_speed) -> Bus Creator/1

== system HEV_Simu_V1_1b/Controller/CAN_Variant/VNT_Level_2_CAN/NAVI/NAVI_CAN_Tx ==
  note: CAN transmit
  note: Navigation
  NAVI_InfoCAN_Tx_Apli : Inport
  Bus Creator1 : BusCreator  Inputs=1
  Bus Selector3 : BusSelector  OutputSignals=NAVI_Home_around_status,NAVI_Road_information
  NAVI_InfoCAN Pack : canmsglib/CAN Pack  CANdbFile=HEV_CANDB.dbc  MsgList=NAVI_InfoCAN_Tx  MsgName=NAVI_InfoCAN_Tx  MsgIDType=Extended (29-bit identifier)  MsgIdentifier=218083356  MsgLength=8  SignalInfo=NAVI_Home_around_status$16$16$1$2$1$0$1$0$0$65535$#NAVI_Road_information$0$16$1$2$1$0$1$0$0$65535$#  NSignals=2  StartBits=str2num('[int32(16);int32(0)]')  SignalSizes=str2num('[int32(16);int32(16)]')  ByteOrders=str2num('[int32(1);int32(1)]')  DataTypes=str2num('[int32(2);int32(2)]')  MultiplexTypes=str2num('[int32(1);int32(1)]')  MultiplexValues=str2num('[double(0);double(0)]')  Factors=str2num('[double(1);double(1)]')  Offsets=str2num('[double(0);double(0)]')  Minimums=str2num('[double(0);double(0)]')  Maximums=str2num('[double(65535);double(65535)]')  Remote=off  ApplyMinMax=off  BusOutput=off
      settings: AttributesFormatString=<CANdbFile = %<CANdbFile>>  SourceProductName=Simulink Real-Time  SourceProductBaseCode=XP  DataFormat=CANdb specified signals
  NAVI_InfoCAN Transmit : canlib/CAN Transmit  BlockHandle=1319.0001  DeviceMenu=MathWorks Virtual 1 (Channel 1)  Device=MathWorks Virtual 1 (Channel 1)  ObjConstructor=canChannel('MathWorks','Virtual 1',1)  EnablePeriodicTransmit=on  MessagePeriod=0.1
      settings: AttributesFormatString=<MessagePeriod = %<MessagePeriod>>  SourceProductName=Vehicle Network Toolbox  SourceProductBaseCode=VN
  NAVI_InfoCAN_Tx : Outport
  wires:
  Bus Creator1/1 -> NAVI_InfoCAN_Tx/1  "NAVI_InfoCAN_Tx"
  Bus Selector3/1 -> NAVI_InfoCAN Pack/1  "<NAVI_Home_around_status>"
  NAVI_InfoCAN Pack/1 -> NAVI_InfoCAN Transmit/1, Bus Creator1/1  "NAVI_InfoCAN_Tx_0CFFB01C"
  Bus Selector3/2 -> NAVI_InfoCAN Pack/2  "<NAVI_Road_information>"
  NAVI_InfoCAN_Tx_Apli/1 -> Bus Selector3/1

== system HEV_Simu_V1_1b/Controller/CAN_Variant/VNT_Level_2_CAN/Radar/Radar_CAN_Rx ==
  note: Function of CAN receive
      | ・CAN message selection
      | ・conversion from CAN signal to CAN application signal with bus object
  note: Radar Detection
  note: CAN receive
  InfoCAN : Inport
  Bus Creator : BusCreator  Inputs=1
  Bus Selector1 : BusSelector  OutputSignals=Gateway_InfoCAN_Tx_0CFFC485
  Radar_InfoCAN Receive : canlib/CAN Receive  BlockHandle=1401.0001  DeviceMenu=MathWorks Virtual 1 (Channel 1)  Device=MathWorks Virtual 1 (Channel 1)  ObjConstructor=canChannel('MathWorks','Virtual 1',1)  EnableStandardIDsFilter=off  StandardIDs=0  EnableExtendedIDsFilter=off  ExtendedIDs=0  SampleTime=0.1  MsgsPerTimestep=all  StdIDsCombo=Allow all  ExtIDsCombo=Allow all  InternalFilterUpdateStatus=on  BusOutput=off
      settings: AttributesFormatString=<SampleTime = %<SampleTime>>  SourceProductName=Vehicle Network Toolbox  SourceProductBaseCode=VN
  Radar_InfoCAN_Receive_100ms : Subsystem
  Rate Transition1 : RateTransition  Deterministic=off
      settings: AttributesFormatString=<Deterministic=%<Deterministic>>
  Terminator : Terminator
  Radar_InfoCAN_Rx : Outport
  wires:
  Rate Transition1/1 -> Radar_InfoCAN_Rx/1  "Radar_InfoCAN_Rx"
  Bus Creator/1 -> Rate Transition1/1
  InfoCAN/1 -> Bus Selector1/1
  Bus Selector1/1 -> Terminator/1  "<Gateway_InfoCAN_Tx_0CFFC485>"
  Radar_InfoCAN_Receive_100ms/1(BrkCtrl_Vehicle_speed) -> Bus Creator/1
  Radar_InfoCAN Receive/2 -> Radar_InfoCAN_Receive_100ms/1(InfoCAN_Msg)
  Radar_InfoCAN Receive/1 -> Radar_InfoCAN_Receive_100ms/Trigger

== system HEV_Simu_V1_1b/Controller/CAN_Variant/VNT_Level_2_CAN/Radar/Radar_CAN_Tx ==
  note: Radar Detection
  note: CAN transmit
  note: Function of CAN transmit
      | ・conversion fromCAN application signal to signal of CAN message
  Radar_InfoCAN_Tx_Apli : Inport
  Bus Creator1 : BusCreator  Inputs=1
  Bus Selector3 : BusSelector  OutputSignals=Radar_Relative_distance,Radar_Relative_velocity
  Radar_InfoCAN Pack : canmsglib/CAN Pack  CANdbFile=HEV_CANDB.dbc  MsgList=Radar_InfoCAN_Tx  MsgName=Radar_InfoCAN_Tx  MsgIDType=Extended (29-bit identifier)  MsgIdentifier=218038400  MsgLength=8  SignalInfo=Radar_Relative_distance$0$16$1$2$1$0$1.000000e-02$0$0$500$#Radar_Relative_velocity$16$16$1$1$1$0$1.000000e-02$0$-50$50$#  NSignals=2  StartBits=str2num('[int32(0);int32(16)]')  SignalSizes=str2num('[int32(16);int32(16)]')  ByteOrders=str2num('[int32(1);int32(1)]')  DataTypes=str2num('[int32(2);int32(1)]')  MultiplexTypes=str2num('[int32(1);int32(1)]')  MultiplexValues=str2num('[double(0);double(0)]')  Factors=str2num('[double(1.000000e-02);double(1.000000e-02)]')  Offsets=str2num('[double(0);double(0)]')  Minimums=str2num('[double(0);double(-50)]')  Maximums=str2num('[double(500);double(50)]')  Remote=off  ApplyMinMax=off  BusOutput=off
      settings: AttributesFormatString=<CANdbFile = %<CANdbFile>>  SourceProductName=Simulink Real-Time  SourceProductBaseCode=XP  DataFormat=CANdb specified signals
  Radar_InfoCAN Transmit : canlib/CAN Transmit  BlockHandle=1429.0001  DeviceMenu=MathWorks Virtual 1 (Channel 1)  Device=MathWorks Virtual 1 (Channel 1)  ObjConstructor=canChannel('MathWorks','Virtual 1',1)  EnablePeriodicTransmit=on  MessagePeriod=0.1
      settings: AttributesFormatString=<MessagePeriod = %<MessagePeriod>>  SourceProductName=Vehicle Network Toolbox  SourceProductBaseCode=VN
  Radar_InfoCAN_Tx : Outport
  wires:
  Bus Creator1/1 -> Radar_InfoCAN_Tx/1  "Radar_InfoCAN_Tx"
  Radar_InfoCAN_Tx_Apli/1 -> Bus Selector3/1
  Radar_InfoCAN Pack/1 -> Bus Creator1/1, Radar_InfoCAN Transmit/1  "Radar_InfoCAN_Tx_0CFF0080"
  Bus Selector3/2 -> Radar_InfoCAN Pack/2  "<Radar_Relative_velocity>"
  Bus Selector3/1 -> Radar_InfoCAN Pack/1  "<Radar_Relative_distance>"

== system HEV_Simu_V1_1b/Controller/CAN_Variant/VNT_Level_2_CAN/Steer_Ctrl/SteerCtrl_VehCAN Tx ==
  note: Steering Control
  note: Function of CAN transmit
      | ・conversion fromCAN application signal to signal of CAN message
  note: CAN transmit
  SteerCtrl_VehCAN_Tx_Apli : Inport
  Bus Creator1 : BusCreator  Inputs=1
  Bus Selector1 : BusSelector  OutputSignals=StrgCtrl_Steer_angle
  SteerCtrl_VehCAN Pack : canmsglib/CAN Pack  CANdbFile=HEV_CANDB.dbc  MsgList=SteerCtrl_VehCAN_Tx  MsgName=SteerCtrl_VehCAN_Tx  MsgIDType=Extended (29-bit identifier)  MsgIdentifier=218066963  MsgLength=8  SignalInfo=StrgCtrl_Steer_angle$0$16$1$1$1$0$3.125000e-02$0$-720$720$#  NSignals=1  StartBits=str2num('[int32(0)]')  SignalSizes=str2num('[int32(16)]')  ByteOrders=str2num('[int32(1)]')  DataTypes=str2num('[int32(1)]')  MultiplexTypes=str2num('[int32(1)]')  MultiplexValues=str2num('[double(0)]')  Factors=str2num('[double(3.125000e-02)]')  Offsets=str2num('[double(0)]')  Minimums=str2num('[double(-720)]')  Maximums=str2num('[double(720)]')  Remote=off  ApplyMinMax=off  BusOutput=off
      settings: AttributesFormatString=<CANdbFile = %<CANdbFile>>  SourceProductName=Simulink Real-Time  SourceProductBaseCode=XP  DataFormat=CANdb specified signals
  SteerCtrl_VehCAN Transmit : canlib/CAN Transmit  BlockHandle=1459.0001  DeviceMenu=MathWorks Virtual 1 (Channel 1)  Device=MathWorks Virtual 1 (Channel 1)  ObjConstructor=canChannel('MathWorks','Virtual 1',1)  EnablePeriodicTransmit=on  MessagePeriod=0.05
      settings: AttributesFormatString=<MessagePeriod = %<MessagePeriod>>  SourceProductName=Vehicle Network Toolbox  SourceProductBaseCode=VN
  SteerCtrl_VehCAN_Tx : Outport
  wires:
  SteerCtrl_VehCAN Pack/1 -> SteerCtrl_VehCAN Transmit/1, Bus Creator1/1  "SteerCtrl_VehCAN_Tx_0CFF7013"
  Bus Selector1/1 -> SteerCtrl_VehCAN Pack/1  "<StrgCtrl_Steer_angle>"
  SteerCtrl_VehCAN_Tx_Apli/1 -> Bus Selector1/1
  Bus Creator1/1 -> SteerCtrl_VehCAN_Tx/1  "SteerCtrl_VehCAN_Tx"

== system HEV_Simu_V1_1b/Controller/CAN_Variant/VNT_Level_2_CAN/Steer_Ctrl/SteerCtrl_VehCAN_Rx ==
  note: Steering Control
  note: Function of CAN receive
      | ・CAN message selection
      | ・conversion from CAN signal to CAN application signal with bus object
  note: CAN receive
  VehCAN : Inport
  Bus Creator : BusCreator  Inputs=1
  Bus Selector7 : BusSelector  OutputSignals=BrakeCtrl_VehCAN_Tx_0CFF600B
  Rate Transition1 : RateTransition  Deterministic=off
      settings: AttributesFormatString=<Deterministic=%<Deterministic>>
  SteerCtrl_VehCAN Receive : canlib/CAN Receive  BlockHandle=1475.0001  DeviceMenu=MathWorks Virtual 1 (Channel 1)  Device=MathWorks Virtual 1 (Channel 1)  ObjConstructor=canChannel('MathWorks','Virtual 1',1)  EnableStandardIDsFilter=off  StandardIDs=0  EnableExtendedIDsFilter=off  ExtendedIDs=0  SampleTime=0.05  MsgsPerTimestep=all  StdIDsCombo=Allow all  ExtIDsCombo=Allow all  InternalFilterUpdateStatus=on  BusOutput=off
      settings: AttributesFormatString=<SampleTime = %<SampleTime>>  SourceProductName=Vehicle Network Toolbox  SourceProductBaseCode=VN
  SteerCtrl_VehCAN_Receive50ms : Subsystem
  Terminator : Terminator
  SteerCtrl_VehCAN_Rx : Outport
  wires:
  VehCAN/1 -> Bus Selector7/1
  Bus Creator/1 -> Rate Transition1/1
  Rate Transition1/1 -> SteerCtrl_VehCAN_Rx/1  "SteerCtrl_VehCAN_Rx"
  Bus Selector7/1 -> Terminator/1  "<BrakeCtrl_VehCAN_Tx_0CFF600B>"
  SteerCtrl_VehCAN_Receive50ms/1(BrkCtrl_Vehicle_speed) -> Bus Creator/1
  SteerCtrl_VehCAN Receive/1 -> SteerCtrl_VehCAN_Receive50ms/Trigger
  SteerCtrl_VehCAN Receive/2 -> SteerCtrl_VehCAN_Receive50ms/1(VehCAN_Msg)

== system HEV_Simu_V1_1b/Controller/CAN_Variant/VNT_Level_2_CAN/Transms_Ctrl/TransmCtrl_PwtrCAN Tx ==
  note: Function of CAN transmit
      | ・conversion fromCAN application signal to signal of CAN message
  note: Transmission Control
  note: CAN transmit
  TransmCtrl_PwtrCAN_Tx_Apli : Inport
  Bus Creator1 : BusCreator  Inputs=1
  Bus Selector2 : BusSelector  OutputSignals=TmCtrl_Clutch_position,TmCtrl_Gear_position
  TransmCtrl_PwtrCAN Pack : canmsglib/CAN Pack  CANdbFile=HEV_CANDB.dbc  MsgList=TransmCtrl_PwtrCAN_Tx  MsgName=TransmCtrl_PwtrCAN_Tx  MsgIDType=Extended (29-bit identifier)  MsgIdentifier=218054659  MsgLength=8  SignalInfo=TmCtrl_Clutch_position$0$8$1$2$1$0$1.000000e-02$0$0$1$#TmCtrl_Gear_position$8$8$1$2$1$0$1$0$0$5$#  NSignals=2  StartBits=str2num('[int32(0);int32(8)]')  SignalSizes=str2num('[int32(8);int32(8)]')  ByteOrders=str2num('[int32(1);int32(1)]')  DataTypes=str2num('[int32(2);int32(2)]')  MultiplexTypes=str2num('[int32(1);int32(1)]')  MultiplexValues=str2num('[double(0);double(0)]')  Factors=str2num('[double(1.000000e-02);double(1)]')  Offsets=str2num('[double(0);double(0)]')  Minimums=str2num('[double(0);double(0)]')  Maximums=str2num('[double(1);double(5)]')  Remote=off  ApplyMinMax=off  BusOutput=off
      settings: AttributesFormatString=<CANdbFile = %<CANdbFile>>  SourceProductName=Simulink Real-Time  SourceProductBaseCode=XP  DataFormat=CANdb specified signals
  TransmCtrl_PwtrCAN Transmit : canlib/CAN Transmit  BlockHandle=1517.0001  DeviceMenu=MathWorks Virtual 1 (Channel 1)  Device=MathWorks Virtual 1 (Channel 1)  ObjConstructor=canChannel('MathWorks','Virtual 1',1)  EnablePeriodicTransmit=on  MessagePeriod=0.01
      settings: AttributesFormatString=<MessagePeriod = %<MessagePeriod>>  SourceProductName=Vehicle Network Toolbox  SourceProductBaseCode=VN
  TransmCtrl_PwtrCAN_Tx : Outport
  wires:
  TransmCtrl_PwtrCAN_Tx_Apli/1 -> Bus Selector2/1
  TransmCtrl_PwtrCAN Pack/1 -> Bus Creator1/1  "TransmCtrl_PwtrCAN_Tx_0CFF4003"
  Bus Creator1/1 -> TransmCtrl_PwtrCAN Transmit/1, TransmCtrl_PwtrCAN_Tx/1  "TransmCtrl_PwtrCAN_Tx"
  Bus Selector2/2 -> TransmCtrl_PwtrCAN Pack/2  "<TmCtrl_Gear_position>"
  Bus Selector2/1 -> TransmCtrl_PwtrCAN Pack/1  "<TmCtrl_Clutch_position>"

== system HEV_Simu_V1_1b/Controller/CAN_Variant/VNT_Level_2_CAN/Transms_Ctrl/TransmCtrl_PwtrCAN_Rx ==
  note: Transmission Control
  note: Function of CAN receive
      | ・CAN message selection
      | ・conversion from CAN signal to CAN application signal with bus object
  note: CAN receive
  PwtrCAN : Inport
  Bus Creator6 : BusCreator  Inputs=2
  Bus Selector3 : BusSelector  OutputSignals=EngineCtrl_PwtrCAN_Tx_0CFF3000
  Bus Selector7 : BusSelector  OutputSignals=Gateway_PwtrCAN_Tx_0CFFC385
  Rate Transition1 : RateTransition  Deterministic=off
      settings: AttributesFormatString=<Deterministic=%<Deterministic>>
  Terminator : Terminator
  Terminator1 : Terminator
  TransmCtrl_PwtrCAN Receive : canlib/CAN Receive  BlockHandle=1537.0001  DeviceMenu=MathWorks Virtual 1 (Channel 1)  Device=MathWorks Virtual 1 (Channel 1)  ObjConstructor=canChannel('MathWorks','Virtual 1',1)  EnableStandardIDsFilter=off  StandardIDs=0  EnableExtendedIDsFilter=off  ExtendedIDs=0  SampleTime=0.01  MsgsPerTimestep=all  StdIDsCombo=Allow all  ExtIDsCombo=Allow all  InternalFilterUpdateStatus=on  BusOutput=off
      settings: AttributesFormatString=<SampleTime = %<SampleTime>>  SourceProductName=Vehicle Network Toolbox  SourceProductBaseCode=VN
  TransmCtrl_PwtrCAN_Receive_10ms : Subsystem
  TransmCtrl_PwtrCAN_Rx : Outport
  wires:
  PwtrCAN/1 -> Bus Selector3/1, Bus Selector7/1
  Rate Transition1/1 -> TransmCtrl_PwtrCAN_Rx/1  "TransmCtrl_PwtrCAN_Rx"
  Bus Creator6/1 -> Rate Transition1/1
  Bus Selector7/1 -> Terminator/1  "<Gateway_PwtrCAN_Tx_0CFFC385>"
  Bus Selector3/1 -> Terminator1/1  "<EngineCtrl_PwtrCAN_Tx_0CFF3000>"
  TransmCtrl_PwtrCAN_Receive_10ms/1(BrkCtrl_Vehicle_speed) -> Bus Creator6/1
  TransmCtrl_PwtrCAN_Receive_10ms/2(EngCtrl_Engine_speed) -> Bus Creator6/2
  TransmCtrl_PwtrCAN Receive/1 -> TransmCtrl_PwtrCAN_Receive_10ms/Trigger
  TransmCtrl_PwtrCAN Receive/2 -> TransmCtrl_PwtrCAN_Receive_10ms/1(PwtrCAN_Msg)
